simulink model "Assignment_5_Silkey"  (R2018b)
settings: Solver=VariableStepAuto  StartTime=0.0  StopTime=1  RelTol=1e-3
undefined symbols (not defined in the file): sigbuilder_block
libraries: powerlib x27, simulink x4, powerlib_meascontrol x3, peRmsMeasurement x2
settings Model: Creator=Marmik  LastModifiedBy=jasil

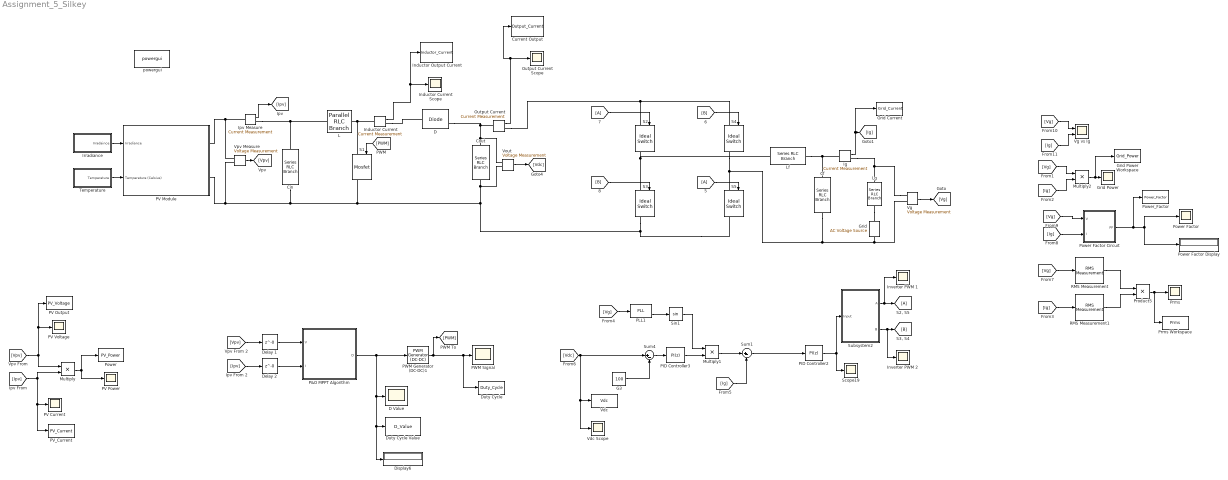
== system Assignment_5_Silkey ==
  Cf : powerlib/Elements/Series RLC Branch  LConnTagsString=__new0  RConnTagsString=__new0  BranchType=RC  Resistance=70e-3  Inductance=1e-3  SetiL0=off  InitialCurrent=0  Capacitance=10e-12  Setx0=off  InitialVoltage=0  Measurements=None
  Cin : powerlib/Elements/Series RLC Branch  LConnTagsString=__new0  RConnTagsString=__new0  BranchType=C  Resistance=1  Inductance=1e-3  SetiL0=off  InitialCurrent=0  Capacitance=1e-3  Setx0=off  InitialVoltage=0  Measurements=None
  Cout : powerlib/Elements/Series RLC Branch  LConnTagsString=__new0  RConnTagsString=__new0  BranchType=C  Resistance=0.1  Inductance=1e-3  SetiL0=off  InitialCurrent=0  Capacitance=1e-3  Setx0=off  InitialVoltage=0  Measurements=None
  Current Output : ToWorkspace  VariableName=Output_Current  SaveFormat=Timeseries  SampleTime=-1
  D : powerlib/Power Electronics/Diode  Ron=0.001  Lon=0  Vf=0  IC=0  UseSnubber=0  Rs=500  Cs=250e-9  Measurements=on
  D Value : Scope
  Delay 1 : Delay  DelayLength=0  SampleTime=0.01
  Delay 2 : Delay  DelayLength=0  SampleTime=0.01
  Display6 : Display
  Duty Cycle : ToWorkspace  VariableName=Duty_Cycle  SaveFormat=Timeseries  SampleTime=-1
  Duty Cycle Value : ToWorkspace  VariableName=D_Value  SaveFormat=Timeseries  SampleTime=-1
  G3 : Constant  Value=100
  Grid : powerlib/Electrical Sources/AC Voltage Source  Amplitude=42.43  Phase=0  Frequency=60  SampleTime=0  Measurements=None  BusType=swing  Pref=10e3  Qref=0  Qmin=-inf  Qmax=+inf
  Grid Current : ToWorkspace  VariableName=Grid_Current  SaveFormat=Timeseries  SampleTime=-1
  Grid Power : Scope
  Grid Power Workspace : ToWorkspace  VariableName=Grid_Power  SaveFormat=Timeseries  SampleTime=-1
  Ig : powerlib/Measurements/Current Measurement  PhasorSimulation=off  OutputType=Complex  PSBequivalent=0
  Inductor Current : powerlib/Measurements/Current Measurement  PhasorSimulation=off  OutputType=Complex  PSBequivalent=0
  Inductor Current Scope : Scope
  Inductor Output Current : ToWorkspace  VariableName=Inductor_Current  SaveFormat=Timeseries  SampleTime=-1
  Inverter PWM 1 : Scope
  Inverter PWM 2 : Scope
  Ipv Measure : powerlib/Measurements/Current Measurement  PhasorSimulation=off  OutputType=Complex  PSBequivalent=0
  Irradiance : Subsystem  Tag=STV Subsys  LoadFcn=sigbuilder_block('load');  StartFcn=sigbuilder_block('start');  StopFcn=sigbuilder_block('stop');  ClipboardFcn=sigbuilder_block('clipboard');  mask(Sigbuilder block){tuvar=[0:10]}
      mask help: Simulink:masks:SigbuilderBlock_MD
      mask init:
      | if ~strcmp(get_param(bdroot(gcbh),'SimulationStatus'),'stopped') tuvar = sigbuilder_block('maskInit'); end
      settings: CopyFcn=sigbuilder_block('copy');  DeleteFcn=sigbuilder_block('delete');  ModelCloseFcn=sigbuilder_block('modelClose');  PreSaveFcn=sigbuilder_block('preSave');  PauseFcn=sigbuilder_block('pause');  ContinueFcn=sigbuilder_block('continue');  NameChangeFcn=sigbuilder_block('namechange');  OpenFcn=sigbuilder_block('open',[437.6 153 550.4 359.25 ]);  CloseFcn=sigbuilder_block('close');
      mask Display: plot(0, 0, 100, 100,[2, 2, 32, 32, 2], [68, 8, 8, 68, 68],[32, 2], [38, 38], [32, 19, 2],[53, 60, 44], [32, 17, 17, 2],[16, 16, 31, 31]);txt = getActiveGroup(gcbh);text(2, 100, txt,'verticalAlignment', 'top');
  L : powerlib/Elements/Parallel RLC Branch  LConnTagsString=a  RConnTagsString=__new0  BranchType=L  Resistance=1  Inductance=35e-3  SetiL0=off  InitialCurrent=0  Capacitance=1e-6  Setx0=off  InitialVoltage=0  Measurements=None
  Lf : powerlib/Elements/Series RLC Branch  LConnTagsString=__new0  RConnTagsString=__new0  BranchType=RL  Resistance=70e-3  Inductance=10e-3  SetiL0=off  InitialCurrent=0  Capacitance=1e-6  Setx0=off  InitialVoltage=0  Measurements=None
  Lg : powerlib/Elements/Series RLC Branch  LConnTagsString=__new0  RConnTagsString=__new0  BranchType=RL  Resistance=10e-3  Inductance=2e-6  SetiL0=off  InitialCurrent=0  Capacitance=1e-6  Setx0=off  InitialVoltage=0  Measurements=None
  Multiply : Product
  Multiply1 : Product
  Multiply2 : Product
  Output Current : powerlib/Measurements/Current Measurement  PhasorSimulation=off  OutputType=Complex  PSBequivalent=0
  Output Current Scope : Scope
  P&O MPPT Algorithm : MATLAB Function  TreatAsAtomicUnit=on
  PID Controller2 : simulink/Continuous/PID Controller  Controller=PI  Form=Parallel  TimeDomain=Discrete-time  SampleTime=-1  IntegratorMethod=Forward Euler  FilterMethod=Forward Euler  ControllerParametersSource=internal  P=1  I=1  D=0.01  UseFilter=on  N=100  TunerSelectOption=Transfer Function Based (PID Tuner App)  InitialConditionSource=internal  InitialConditionForIntegrator=0  InitialConditionForFilter=0  DifferentiatorICPrevScaledInput=0  ExternalReset=none  TrackingMode=off  Kt=1  LimitOutput=off  UpperSaturationLimit=inf  LowerSaturationLimit=-inf  LinearizeAsGain=on  AntiWindupMode=none  Kb=1  POutMin=[]  POutMax=[]  IOutMin=[]  IOutMax=[]  DOutMin=[]  DOutMax=[]  NOutMin=[]  NOutMax=[]  SumOutMin=[]  SumOutMax=[]  SaturationOutMin=[]  SaturationOutMax=[]  PParamMin=[]  PParamMax=[]  IParamMin=[]  IParamMax=[]  DParamMin=[]  DParamMax=[]  NParamMin=[]  NParamMax=[]  KbParamMin=[]  KbParamMax=[]  KtParamMin=[]  KtParamMax=[]  KbOutMin=[]  KbOutMax=[]  KtOutMin=[]  KtOutMax=[]  IntegratorOutMin=[]  IntegratorOutMax=[]  FilterOutMin=[]  FilterOutMax=[]  SumI1OutMin=[]  SumI1OutMax=[]  SumI2OutMin=[]  SumI2OutMax=[]  SumI3OutMin=[]  SumI3OutMax=[]  SumI4OutMin=[]  SumI4OutMax=[]  SumDOutMin=[]  SumDOutMax=[]  DifferentiatorOutMin=[]  DifferentiatorOutMax=[]  FilterDiffOutCoefMin=[]  FilterDiffOutCoefMax=[]  ReciprocalOutMin=[]  ReciprocalOutMax=[]  SumDenOutMin=[]  SumDenOutMax=[]  SumNumOutMin=[]  SumNumOutMax=[]  DivideOutMin=[]  DivideOutMax=[]  IntegratorContinuousStateAttributes=''  IntegratorStateMustResolveToSignalObject=off  IntegratorRTWStateStorageClass=Auto  FilterContinuousStateAttributes=''  FilterStateMustResolveToSignalObject=off  FilterRTWStateStorageClass=Auto  ParallelPVariant=InternalParameters  IdealPVariant=Disabled  IVariant=InternalParameters  DVariant=Disabled  IntegratorVariant=Discrete  SatVariant=Disabled  AWVariant=Passthrough  PCopyVariant=Disabled  TRVariant=Disabled  FdbkBlocksVariant=Forward  IdealPFdbkVariant=Disabled  SatFdbkVariant=Disabled  DerivativeFilterVariant=Disabled  NVariant=Disabled  NCopyVariant=Disabled_SignalSpec  FilterICVariant=Disabled  IntegratorICVariant=InternalICs  ExternalResetVariant=Disabled  TRSumVariant=Passthrough  SumFdbkVariant=Disabled  SumVariant=Sum_PI
  PID Controller3 : simulink/Continuous/PID Controller  Controller=PI  Form=Parallel  TimeDomain=Discrete-time  SampleTime=-1  IntegratorMethod=Forward Euler  FilterMethod=Forward Euler  ControllerParametersSource=internal  P=0.0625  I=0.625  D=0.01  UseFilter=on  N=100  TunerSelectOption=Transfer Function Based (PID Tuner App)  InitialConditionSource=internal  InitialConditionForIntegrator=0  InitialConditionForFilter=0  DifferentiatorICPrevScaledInput=0  ExternalReset=none  TrackingMode=off  Kt=1  LimitOutput=off  UpperSaturationLimit=inf  LowerSaturationLimit=-inf  LinearizeAsGain=on  AntiWindupMode=none  Kb=1  POutMin=[]  POutMax=[]  IOutMin=[]  IOutMax=[]  DOutMin=[]  DOutMax=[]  NOutMin=[]  NOutMax=[]  SumOutMin=[]  SumOutMax=[]  SaturationOutMin=[]  SaturationOutMax=[]  PParamMin=[]  PParamMax=[]  IParamMin=[]  IParamMax=[]  DParamMin=[]  DParamMax=[]  NParamMin=[]  NParamMax=[]  KbParamMin=[]  KbParamMax=[]  KtParamMin=[]  KtParamMax=[]  KbOutMin=[]  KbOutMax=[]  KtOutMin=[]  KtOutMax=[]  IntegratorOutMin=[]  IntegratorOutMax=[]  FilterOutMin=[]  FilterOutMax=[]  SumI1OutMin=[]  SumI1OutMax=[]  SumI2OutMin=[]  SumI2OutMax=[]  SumI3OutMin=[]  SumI3OutMax=[]  SumI4OutMin=[]  SumI4OutMax=[]  SumDOutMin=[]  SumDOutMax=[]  DifferentiatorOutMin=[]  DifferentiatorOutMax=[]  FilterDiffOutCoefMin=[]  FilterDiffOutCoefMax=[]  ReciprocalOutMin=[]  ReciprocalOutMax=[]  SumDenOutMin=[]  SumDenOutMax=[]  SumNumOutMin=[]  SumNumOutMax=[]  DivideOutMin=[]  DivideOutMax=[]  IntegratorContinuousStateAttributes=''  IntegratorStateMustResolveToSignalObject=off  IntegratorRTWStateStorageClass=Auto  FilterContinuousStateAttributes=''  FilterStateMustResolveToSignalObject=off  FilterRTWStateStorageClass=Auto  ParallelPVariant=InternalParameters  IdealPVariant=Disabled  IVariant=InternalParameters  DVariant=Disabled  IntegratorVariant=Discrete  SatVariant=Disabled  AWVariant=Passthrough  PCopyVariant=Disabled  TRVariant=Disabled  FdbkBlocksVariant=Forward  IdealPFdbkVariant=Disabled  SatFdbkVariant=Disabled  DerivativeFilterVariant=Disabled  NVariant=Disabled  NCopyVariant=Disabled_SignalSpec  FilterICVariant=Disabled  IntegratorICVariant=InternalICs  ExternalResetVariant=Disabled  TRSumVariant=Passthrough  SumFdbkVariant=Disabled  SumVariant=Sum_PI
  PLL1 : powerlib_meascontrol/PLL/PLL  Fmin=45  Par_Init=[0, 60]  ParK=[180, 3200, 1]  TcD=1e-4  MaxRateChangeFreq=12  FilterCutOffFreq=25  Ts=1e-6  AGC=on
      settings: SourceProductName=Simscape Power Systems  SourceProductBaseCode=PS
  PV Current : Scope
  PV Module : Subsystem
  PV Output : ToWorkspace  VariableName=PV_Voltage  SaveFormat=Timeseries  SampleTime=-1
  PV Power : Scope
  PV Voltage : Scope
  PV_Current : ToWorkspace  VariableName=PV_Current  SaveFormat=Timeseries  SampleTime=-1
  PWM Generator (DC-DC)1 : powerlib_meascontrol/Pulse & Signal Generators/PWM Generator (DC-DC)  Fsw=30000  Ts=0
  PWM Signal : Scope
  Power : ToWorkspace  VariableName=PV_Power  SaveFormat=Timeseries  SampleTime=-1
  Power Factor : Scope
  Power Factor Circuit : Subsystem
  Power Factor Display : Display
  Power_Factor : ToWorkspace  VariableName=Power_Factor  SaveFormat=Timeseries  SampleTime=-1
  "Prms " : Scope
  Prms Workspace : ToWorkspace  VariableName=Prms  SaveFormat=Timeseries  SampleTime=-1
  Product5 : Product
  RMS Measurement : peRmsMeasurement/RMS Measurement  LabelModeActiveChoice=Total  F=60  SpecifyHarmonics=off  K=[0 1 2]  Ts=0
  RMS Measurement1 : peRmsMeasurement/RMS Measurement  LabelModeActiveChoice=Total  F=60  SpecifyHarmonics=off  K=[0 1 2]  Ts=0
  S1 : powerlib/Power Electronics/Mosfet  Ron=0.1  Lon=0  Rd=0.01  Vfd=0  IC=0  Rs=1e5  Cs=inf  Measurements=on
  S{2..5} (4 alike) : powerlib/Power Electronics/Ideal Switch  Ron=0.001  Lon=0  IC=0  Rs=1e5  Cs=inf  Measurements=on
  Scope19 : Scope
  Sin1 : Trigonometry
  Subsystem2 : Subsystem
  Sum1 : Sum  Inputs=|+-
  Sum4 : Sum  Inputs=|+-
  Temperature : Subsystem  Tag=STV Subsys  LoadFcn=sigbuilder_block('load');  StartFcn=sigbuilder_block('start');  StopFcn=sigbuilder_block('stop');  ClipboardFcn=sigbuilder_block('clipboard');  mask(Sigbuilder block){tuvar=[0:10]}
      mask help: Simulink:masks:SigbuilderBlock_MD
      mask init:
      | if ~strcmp(get_param(bdroot(gcbh),'SimulationStatus'),'stopped') tuvar = sigbuilder_block('maskInit'); end
      settings: CopyFcn=sigbuilder_block('copy');  DeleteFcn=sigbuilder_block('delete');  ModelCloseFcn=sigbuilder_block('modelClose');  PreSaveFcn=sigbuilder_block('preSave');  PauseFcn=sigbuilder_block('pause');  ContinueFcn=sigbuilder_block('continue');  NameChangeFcn=sigbuilder_block('namechange');  OpenFcn=sigbuilder_block('open',[437.6 153 550.4 359.25 ]);  CloseFcn=sigbuilder_block('close');
      mask Display: plot(0, 0, 100, 100,[2, 2, 32, 32, 2], [68, 8, 8, 68, 68],[32, 2], [38, 38], [32, 19, 2],[53, 60, 44], [32, 17, 17, 2],[16, 16, 31, 31]);txt = getActiveGroup(gcbh);text(2, 100, txt,'verticalAlignment', 'top');
  Vdc : ToWorkspace  VariableName=Vdc  SaveFormat=Timeseries  SampleTime=-1
  Vdc Scope : Scope
  Vg : powerlib/Measurements/Voltage Measurement  PhasorSimulation=off  OutputType=Complex  PSBequivalent=0
  Vg vs Ig : Scope  NumInputPorts=2
  Vout : powerlib/Measurements/Voltage Measurement  PhasorSimulation=off  OutputType=Complex  PSBequivalent=0
  Vpv Measure : powerlib/Measurements/Voltage Measurement  PhasorSimulation=off  OutputType=Complex  PSBequivalent=0
  powergui : powerlib/powergui  Priority=1  SimulationMode=Discrete  SampleTime=1e-6  frequency=60  Iterations=50  frequencyindice=0  Pbase=100e6  ErrMax=1e-4  UnitsV=kV  UnitsW=MW  buscounter=0  FunctionMessages=off  echomessages=off  EnableUseOfTLC=off  CurrentSourceSwitches=off  DisableSnubberDevices=off  DisableRonSwitches=off  DisableVfSwitches=off  DisplayEquations=off  SolverType=Tustin/Backward Euler (TBE)  Interpol=off  ExternalGateDelay=off  methode=off  Ts=100  x0status=blocks  SPID=off  SwTol=0  HookPort=off  RestoreLinks=warning  ResistiveCurrentMeasurement=off  Frange=[0:2:500]  Ylog=off  Xlog=on  ShowGrid=off  save=off  variable=ZData  structure=0  ZoomFFT=off  StartTime=0.0  cycles=1  DisplayStyle=1  fundamental=60  FreqAxis=off  MaxFrequency=1000  frequencyindicesteady=1  RmsSteady=1  display=off
  wires:
  PWM Generator (DC-DC)1/1 -> [PWM], Duty Cycle/1, PWM Signal/1
  Inductor Current/1 -> Inductor Output Current/1, Inductor Current Scope/1
  Vpv Measure/1 -> [Vpv]
  Multiply/1 -> Power/1, PV Power/1
  Ipv Measure/1 -> [Ipv]
  [Vpv] -> Multiply/1, PV Output/1, PV Voltage/1
  [Ipv] -> PV_Current/1, PV Current/1, Multiply/2
  [Ipv] -> Delay 2/1
  [Vpv] -> Delay 1/1
  [PWM] -> S1/1
  Irradiance/1(Irradaince) -> PV Module/1(Irradiance)
  Temperature/1(Temperature) -> PV Module/2(Temperature (Celsius))
  [A] -> S5/1
  Vg/1 -> [Vg]
  Vout/1 -> [Vdc]
  [B] -> S3/1
  [A] -> S2/1
  Output Current/1 -> Current Output/1, Output Current Scope/1
  [B] -> S4/1
  Ig/1 -> Grid Current/1, [Ig]
  Subsystem2/2(B) -> Inverter PWM 2/1, [B]
  [Vdc] -> Vdc/1, Vdc Scope/1, Sum4/1
  [Vg] -> PLL1/1
  Sum4/1 -> PID Controller3/1
  Subsystem2/1(A) -> Inverter PWM 1/1, [A]
  G3/1 -> Sum4/2
  [Ig] -> Sum1/2
  PID Controller3/1 -> Multiply1/2
  PLL1/2 -> Sin1/1
  Multiply1/1 -> Sum1/1
  Sin1/1 -> Multiply1/1
  PID Controller2/1 -> Scope19/1, Subsystem2/1(Input)
  Sum1/1 -> PID Controller2/1
  [Ig] -> Power Factor Circuit/2(I)
  [Vg] -> Power Factor Circuit/1(V)
  Product5/1 -> Prms Workspace/1, "Prms "/1
  [Vg] -> RMS Measurement/1
  Power Factor Circuit/1(PF) -> Power_Factor/1, Power Factor/1, Power Factor Display/1
  [Ig] -> Multiply2/2
  [Vg] -> Vg vs Ig/1
  RMS Measurement/1 -> Product5/1
  [Ig] -> RMS Measurement1/1
  RMS Measurement1/1 -> Product5/2
  [Vg] -> Multiply2/1
  Multiply2/1 -> Grid Power Workspace/1, Grid Power/1
  [Ig] -> Vg vs Ig/2
  Delay 1/1 -> P&O MPPT Algorithm/1(V)
  Delay 2/1 -> P&O MPPT Algorithm/2(I)
  P&O MPPT Algorithm/1(D) -> Display6/1, Duty Cycle Value/1, D Value/1, PWM Generator (DC-DC)1/1
  connections:
  Vpv Measure/LConn1 -- Ipv Measure/LConn1 -- PV Module/RConn1
  Ipv Measure/RConn1 -- L/LConn1 -- Cin/LConn1
  S1/LConn1 -- Inductor Current/LConn1 -- L/RConn1
  Inductor Current/RConn1 -- D/LConn1
  D/RConn1 -- Output Current/LConn1 -- Vout/LConn1 -- Cout/LConn1
  Cf/RConn1 -- S4/RConn1 -- S5/LConn1 -- Grid/LConn1 -- Vg/LConn2
  Cf/LConn1 -- Ig/LConn1 -- Lf/RConn1
  Lf/LConn1 -- S2/RConn1 -- S3/LConn1
  Vg/LConn1 -- Ig/RConn1 -- Lg/LConn1
  Output Current/RConn1 -- S2/LConn1 -- S4/LConn1
  Cin/RConn1 -- Vpv Measure/LConn2 -- PV Module/RConn2 -- S5/RConn1 -- S3/RConn1 -- Vout/LConn2 -- Cout/RConn1 -- S1/RConn1
  Lg/RConn1 -- Grid/RConn1

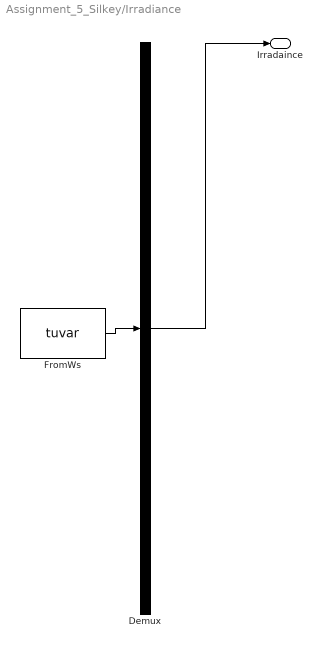
== system Assignment_5_Silkey/Irradiance ==
  Demux : Demux  Tag=STV Demux  Outputs=1
  FromWs : FromWorkspace  Tag=STV FromWs  VariableName=tuvar  SampleTime=0
      SigBuilderData=|
      | common.afterFinalStr = 'Extrapolate'
      | common.sampleTime = 0
      | dataSet.timeRange = [0 1]
      | dataSet.name = 'Input 1'
      | sbobj.Groups.Name = 'Input 1'
      | sbobj.Groups.Signals.Name = 'Irradaince'
      | sbobj.Groups.Signals.XData = [0 0.5 0.5 1]
      | sbobj.Groups.Signals.YData = [1 1 0.5 0.5]
      | sbobj.Groups.TimeRange = [0 1]
  Irradaince : Outport  Tag=STV Outport
  wires:
  Demux/1 -> Irradaince/1
  FromWs/1 -> Demux/1

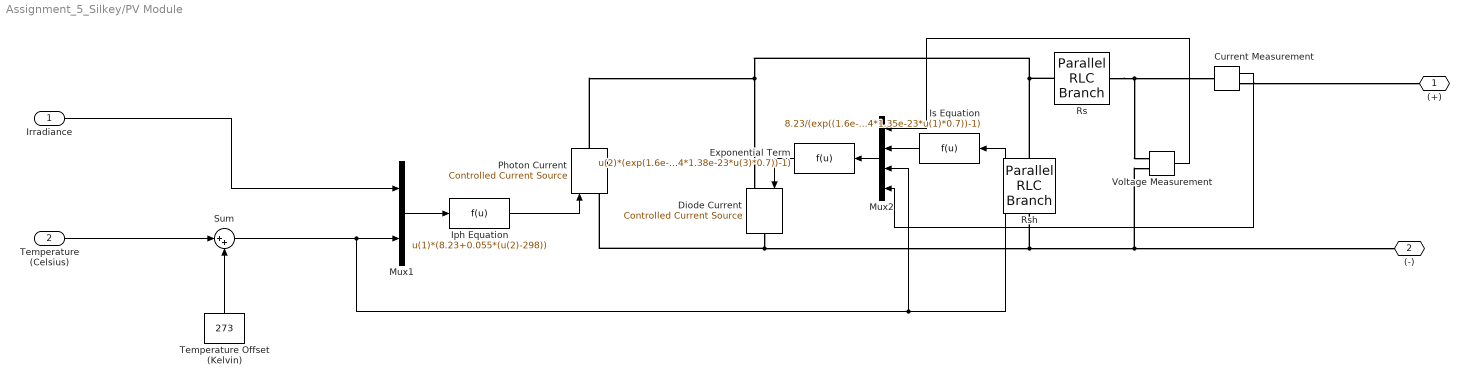
== system Assignment_5_Silkey/PV Module ==
  Irradiance : Inport
  Temperature (Celsius) : Inport  Port=2
  Current Measurement : powerlib/Measurements/Current Measurement  PhasorSimulation=off  OutputType=Complex  PSBequivalent=0
      settings: SourceProductName=Simscape Electrical
  Diode Current : powerlib/Electrical Sources/Controlled Current Source  Initialize=on  Source_Type=AC  Amplitude=0  Phase=0  Frequency=0  Measurements=None
      settings: SourceProductName=Simscape Electrical
  Exponential Term : Fcn  Expr=u(2)*(exp(1.6e-19*(u(1)+u(4)* 0.5272)/(54*1.38e-23*u(3)*0.7))-1)
  Iph Equation : Fcn  Expr=u(1)*(8.23+0.055*(u(2)-298))
  "Is Equation " : Fcn  Expr=8.23/(exp((1.6e-19*(33.5-(0.33*(u(1)-298))))/(54*1.35e-23*u(1)*0.7))-1)
  Mux1 : Mux  Inputs=2
  Mux2 : Mux
  Photon Current : powerlib/Electrical Sources/Controlled Current Source  Initialize=on  Source_Type=AC  Amplitude=0  Phase=0  Frequency=0  Measurements=None
      settings: SourceProductName=Simscape Electrical
  Rs : powerlib/Elements/Parallel RLC Branch  LConnTagsString=a  RConnTagsString=__new0  BranchType=R  Resistance=0.5272  Inductance=1e-3  SetiL0=off  InitialCurrent=0  Capacitance=1e-6  Setx0=off  InitialVoltage=0  Measurements=None
      settings: SourceProductName=Simscape Electrical
  Rsh : powerlib/Elements/Parallel RLC Branch  LConnTagsString=a  RConnTagsString=__new0  BranchType=R  Resistance=332.8212  Inductance=1e-3  SetiL0=off  InitialCurrent=0  Capacitance=1e-6  Setx0=off  InitialVoltage=0  Measurements=None
      settings: SourceProductName=Simscape Electrical
  Sum : Sum  Inputs=|++
  Temperature Offset (Kelvin) : Constant  Value=273
  Voltage Measurement : powerlib/Measurements/Voltage Measurement  PhasorSimulation=off  OutputType=Complex  PSBequivalent=0
      settings: SourceProductName=Simscape Electrical
  (+) : PMIOPort  Side=Right
  (-) : PMIOPort  Port=2  Side=Right
  wires:
  "Is Equation "/1 -> Mux2/2
  Mux2/1 -> Exponential Term/1
  Exponential Term/1 -> Diode Current/1
  Mux1/1 -> Iph Equation/1
  Iph Equation/1 -> Photon Current/1
  Irradiance/1 -> Mux1/1
  Voltage Measurement/1 -> Mux2/1
  Current Measurement/1 -> Mux2/4
  Temperature (Celsius)/1 -> Sum/1
  Temperature Offset (Kelvin)/1 -> Sum/2
  Sum/1 -> Mux1/2, Mux2/3, "Is Equation "/1
  connections:
  Current Measurement/RConn1 -- (+)/RConn1
  Rs/RConn1 -- Current Measurement/LConn1 -- Voltage Measurement/LConn1
  Rsh/RConn1 -- Diode Current/RConn1 -- Photon Current/LConn1 -- (-)/RConn1 -- Voltage Measurement/LConn2
  Rs/LConn1 -- Rsh/LConn1 -- Photon Current/RConn1 -- Diode Current/LConn1

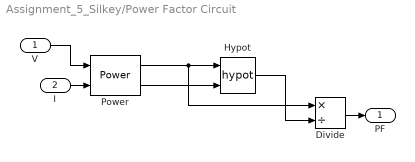
== system Assignment_5_Silkey/Power Factor Circuit ==
  V : Inport
  I : Inport  Port=2
  Divide : Product  Inputs=*/
  Hypot : Math  Operator=hypot  SaturateOnIntegerOverflow=on
  Power : powerlib_meascontrol/Measurements/Power  Freq=60  Vinit=[1, 0]  Iinit=[1, 0]  Ts=1e-6
      settings: SourceProductName=Simscape Power Systems
  PF : Outport
  wires:
  Divide/1 -> PF/1
  Hypot/1 -> Divide/2
  Power/1 -> Hypot/1, Divide/1
  I/1 -> Power/2
  V/1 -> Power/1
  Power/2 -> Hypot/2

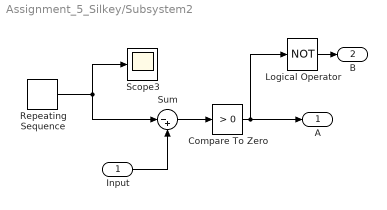
== system Assignment_5_Silkey/Subsystem2 ==
  Input : Inport
  Compare To Zero : simulink/Logic and Bit Operations/Compare To Zero  relop=>  OutDataTypeStr=boolean
  Logical Operator : Logic  Operator=NOT  AllPortsSameDT=off  OutDataTypeStr=boolean
  Repeating Sequence : simulink/Sources/Repeating Sequence  rep_seq_t=[0 1/(4*30000) 3/(4*30000) 1/30000]  rep_seq_y=[0 1 -1 0]
  Scope3 : Scope
  Sum : Sum  Inputs=|-+
  A : Outport
  B : Outport  Port=2
  wires:
  Compare To Zero/1 -> A/1, Logical Operator/1
  Sum/1 -> Compare To Zero/1
  Repeating Sequence/1 -> Sum/1, Scope3/1
  Input/1 -> Sum/2
  Logical Operator/1 -> B/1

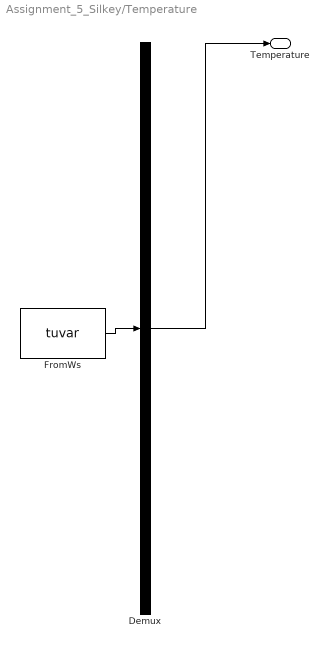
== system Assignment_5_Silkey/Temperature ==
  Demux : Demux  Tag=STV Demux  Outputs=1
  FromWs : FromWorkspace  Tag=STV FromWs  VariableName=tuvar  SampleTime=0
      SigBuilderData=|
      | common.afterFinalStr = 'Extrapolate'
      | common.sampleTime = 0
      | dataSet.timeRange = [0 1]
      | dataSet.name = 'Input 2'
      | sbobj.Groups.Name = 'Input 2'
      | sbobj.Groups.Signals.Name = 'Temperature'
      | sbobj.Groups.Signals.XData = [0 0.5 0.5 1]
      | sbobj.Groups.Signals.YData = [25 25 50 50]
      | sbobj.Groups.TimeRange = [0 1]
  Temperature : Outport  Tag=STV Outport
  wires:
  Demux/1 -> Temperature/1
  FromWs/1 -> Demux/1

== matlab function Assignment_5_Silkey/P&O MPPT Algorithm ==
  data: V input; D output; I input
function D = PandO(V, I)
persistent p_prev;
persistent v_prev;
persistent d_prev; 


if isempty(d_prev)
    d_prev = 0.70;
    v_prev = 33.5;
    p_prev = 0;
end

% Select the change in duty cycle
delta_D = 0.01;

% Set local variables and calculate pv module power 
Vn = V;
In = I;
Pn = Vn*In;

% Increase or decrease duty cycle based on conditions
if ((Pn - p_prev) ~= 0)
    if ((Pn - p_prev) > 0)
        if ((Vn - v_prev) > 0)
            D = d_prev - delta_D;
        else
            D = d_prev + delta_D;
        end
    else
        if ((Vn - v_prev) > 0)
            D = d_prev + delta_D;
        else
            D = d_prev - delta_D;
        end        
    end
else
    D = d_prev;
end
% Update internal values
d_prev = D;
v_prev = Vn;
p_prev = Pn;
